simulink model "B20_ATMD_Earthquake"  (R2020b)
settings: Solver=ode45  StartTime=0.0  StopTime=30  FixedStep=Ts  MaxStep=Ts  MinStep=0.005  RelTol=1e-2
values from neighbouring files (symbols this model uses):
  DoS_on = 0    [main.m]
  EI = 0    [main.m]
  FDI_amp = 300e3    (= 300000)    [main.m]
  FDI_fr = 1/3.5104    (= 0.284867821331)    [main.m]
  FDIon = 1    [main.m]
  K_lqr = lqr(A,B,Q,R)    [main.m]
  MaxF = 2000e3    (= 2000000)    [main.m]
  nx = length(A)    [main.m]
  Sys_con = ss(A,[E B],C,D)    [main.m]
  Sys_unc = ss(A_ref,E_ref,C_ref,DD_ref)    [main.m]
  Ts = 0.01    [main.m]
  TsEarthquake = EQ.time(2)    [main.m]
undefined symbols (not defined in the file or in its folder): discount, j, So, threshold, wg2, zwg
libraries: simulink x43, dspindex x2, eeLuenbergerObserver x1
settings Model: Creator=drsoto  LastModifiedBy=ferch
settings SolverCC: AlgebraicLoopSolver=LineSearch
settings DataIOCC: ReturnWorkspaceOutputs=off
settings DebuggingCC: AlgebraicLoopMsg=none  ArithmeticOperatorsInVariantConditions=warning
settings SFSimCC: SimUseLocalCustomCode=off  CustomCodeUndefinedFunction=UseInterfaceOnly
settings RTWCC: RTWUseLocalCustomCode=off
settings CodeAppCC: StateflowObjectComments=on

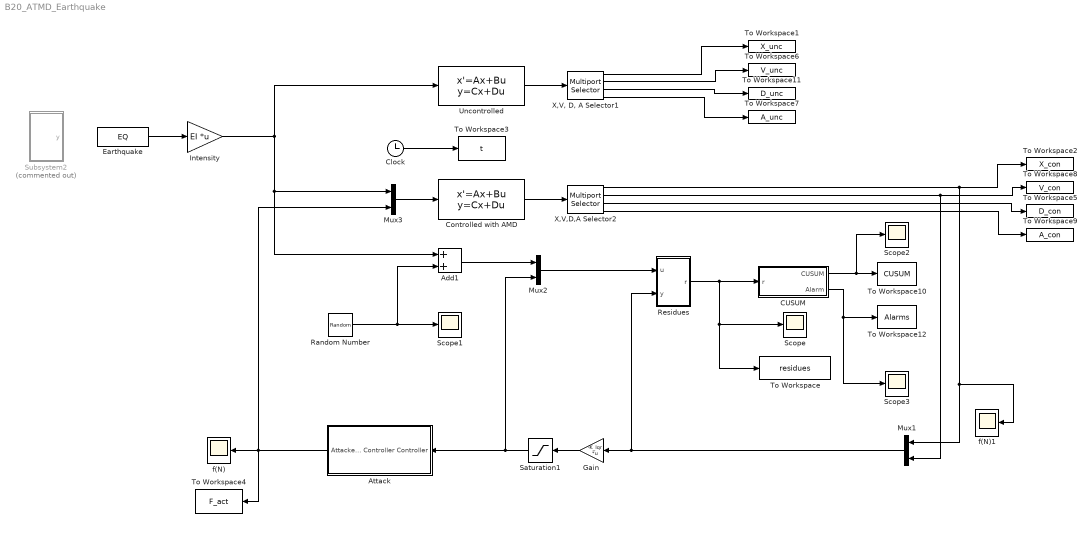
== system B20_ATMD_Earthquake ==
  Add1 : Sum
  Attack : Subsystem
  CUSUM : Subsystem
  Clock : Clock
  Controlled with AMD : StateSpace  A=Sys_con.A  B=Sys_con.B  C=Sys_con.C  D=Sys_con.D  InitialCondition=0
  Earthquake : FromWorkspace  VariableName=EQ  SampleTime=TsEarthquake
  Gain : Gain  Gain=-K_lqr  Multiplication=Matrix(K*u)
  Intensity : Gain  Gain=EI  Multiplication=Matrix(K*u)
  Mux1 : Mux  Inputs=2
  Mux2 : Mux  Inputs=2
  Mux3 : Mux  Inputs=2
  Random Number : RandomNumber  Variance=0.01  Seed=j  SampleTime=Ts
  Residues : Subsystem
  Saturation1 : Saturate  UpperLimit=MaxF  LowerLimit=-MaxF
  Scope{,1..3} (4 alike) : Scope
  Subsystem2 : Subsystem  Commented=on
  To Workspace : ToWorkspace  VariableName=residues  SaveFormat=Timeseries  SampleTime=-1
  To Workspace1 : ToWorkspace  VariableName=X_unc  SampleTime=-1
  To Workspace10 : ToWorkspace  VariableName=CUSUM  SaveFormat=Timeseries  SampleTime=-1
  To Workspace11 : ToWorkspace  VariableName=D_unc  SampleTime=-1
  To Workspace12 : ToWorkspace  VariableName=Alarms  SaveFormat=Timeseries  SampleTime=-1
  To Workspace2 : ToWorkspace  VariableName=X_con  SampleTime=-1
  To Workspace3 : ToWorkspace  VariableName=t  SampleTime=-1
      settings: Save2DSignal=2-D array (concatenate along first dimension)
  To Workspace4 : ToWorkspace  VariableName=F_act  SampleTime=-1
  To Workspace5 : ToWorkspace  VariableName=D_con  SampleTime=-1
  To Workspace6 : ToWorkspace  VariableName=V_unc  SampleTime=-1
  To Workspace7 : ToWorkspace  VariableName=A_unc  SampleTime=-1
  To Workspace8 : ToWorkspace  VariableName=V_con  SampleTime=-1
  To Workspace9 : ToWorkspace  VariableName=A_con  SampleTime=-1
  Uncontrolled : StateSpace  A=Sys_unc.A  B=Sys_unc.B  C=Sys_unc.C  D=Sys_unc.D  InitialCondition=0
  "X,V, D, A Selector1" : dspindex/Multiport Selector  rowsOrCols=Rows  idxCellArray={ 1:n,n+1:2*n,2*n+1:3*n,3*n+1:4*n}  idxErrMode=Clip Index
  X,V,D,A Selector2 : dspindex/Multiport Selector  rowsOrCols=Rows  idxCellArray={ 1:n_amd,n_amd+1:2*n_amd,2*n_amd+1:3*n_amd,3*n_amd+1:4*n_amd}  idxErrMode=Clip Index
  f(N) : Scope
  f(N)1 : Scope
  wires:
  Intensity/1 -> Uncontrolled/1, Mux3/1, Add1/1
  Uncontrolled/1 -> "X,V, D, A Selector1"/1
  Controlled with AMD/1 -> X,V,D,A Selector2/1
  Clock/1 -> To Workspace3/1
  "X,V, D, A Selector1"/2 -> To Workspace6/1
  Mux3/1 -> Controlled with AMD/1
  "X,V, D, A Selector1"/4 -> To Workspace7/1
  "X,V, D, A Selector1"/3 -> To Workspace11/1
  X,V,D,A Selector2/3 -> To Workspace5/1
  X,V,D,A Selector2/4 -> To Workspace9/1
  "X,V, D, A Selector1"/1 -> To Workspace1/1
  X,V,D,A Selector2/1 -> Mux1/1, f(N)1/1, To Workspace2/1
  X,V,D,A Selector2/2 -> To Workspace8/1, Mux1/2
  Gain/1 -> Saturation1/1
  Mux1/1 -> Residues/2(y), Gain/1
  Random Number/1 -> Scope1/1, Add1/2
  Add1/1 -> Mux2/1
  CUSUM/1(CUSUM) -> To Workspace10/1, Scope2/1
  Saturation1/1 -> Mux2/2, Attack/1(Controller)
  Residues/1(r) -> To Workspace/1, Scope/1, CUSUM/1(r)
  Mux2/1 -> Residues/1(u)
  CUSUM/2(Alarm) -> To Workspace12/1, Scope3/1
  Earthquake/1 -> Intensity/1
  Attack/1(Attacked Controller) -> Mux3/2, To Workspace4/1, f(N)/1

== system B20_ATMD_Earthquake/Attack ==
  Controller : Inport
  Constant : Constant  Value=FDIon
  Gain1 : Gain  Gain=1-DoS_on
  Saturation : Saturate  UpperLimit=MaxF  LowerLimit=-MaxF
  Sine Wave : Sin  Amplitude=FDI_amp  Frequency=FDI_fr*2*pi  SampleTime=0
  Switch : Switch  Criteria=u2 > Threshold
  Attacked Controller : Outport
  wires:
  Saturation/1 -> Gain1/1
  Controller/1 -> Switch/3
  Sine Wave/1 -> Switch/1
  Constant/1 -> Switch/2
  Switch/1 -> Saturation/1
  Gain1/1 -> Attacked Controller/1

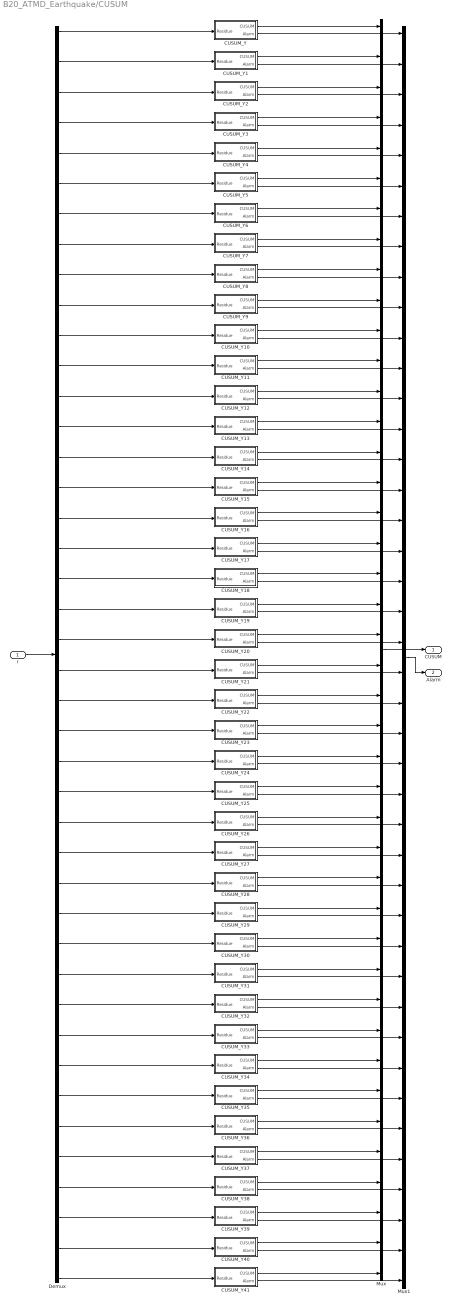
== system B20_ATMD_Earthquake/CUSUM ==
  r : Inport
  CUSUM_Y : Subsystem  mask{i=1}
      mask prompts: i "sensor"
  CUSUM_Y1 : Subsystem  mask{i=2}
      mask prompts: i "sensor"
  CUSUM_Y10 : Subsystem  mask{i=11}
      mask prompts: i "sensor"
  CUSUM_Y11 : Subsystem  mask{i=12}
      mask prompts: i "sensor"
  CUSUM_Y12 : Subsystem  mask{i=13}
      mask prompts: i "sensor"
  CUSUM_Y13 : Subsystem  mask{i=14}
      mask prompts: i "sensor"
  CUSUM_Y14 : Subsystem  mask{i=15}
      mask prompts: i "sensor"
  CUSUM_Y15 : Subsystem  mask{i=16}
      mask prompts: i "sensor"
  CUSUM_Y16 : Subsystem  mask{i=17}
      mask prompts: i "sensor"
  CUSUM_Y17 : Subsystem  mask{i=18}
      mask prompts: i "sensor"
  CUSUM_Y18 : Subsystem  mask{i=19}
      mask prompts: i "sensor"
  CUSUM_Y19 : Subsystem  mask{i=20}
      mask prompts: i "sensor"
  CUSUM_Y2 : Subsystem  mask{i=3}
      mask prompts: i "sensor"
  CUSUM_Y20 : Subsystem  mask{i=21}
      mask prompts: i "sensor"
  CUSUM_Y21 : Subsystem  mask{i=22}
      mask prompts: i "sensor"
  CUSUM_Y22 : Subsystem  mask{i=23}
      mask prompts: i "sensor"
  CUSUM_Y23 : Subsystem  mask{i=24}
      mask prompts: i "sensor"
  CUSUM_Y24 : Subsystem  mask{i=25}
      mask prompts: i "sensor"
  CUSUM_Y25 : Subsystem  mask{i=26}
      mask prompts: i "sensor"
  CUSUM_Y26 : Subsystem  mask{i=27}
      mask prompts: i "sensor"
  CUSUM_Y27 : Subsystem  mask{i=28}
      mask prompts: i "sensor"
  CUSUM_Y28 : Subsystem  mask{i=29}
      mask prompts: i "sensor"
  CUSUM_Y29 : Subsystem  mask{i=30}
      mask prompts: i "sensor"
  CUSUM_Y3 : Subsystem  mask{i=4}
      mask prompts: i "sensor"
  CUSUM_Y30 : Subsystem  mask{i=31}
      mask prompts: i "sensor"
  CUSUM_Y31 : Subsystem  mask{i=31}
      mask prompts: i "sensor"
  CUSUM_Y32 : Subsystem  mask{i=33}
      mask prompts: i "sensor"
  CUSUM_Y33 : Subsystem  mask{i=34}
      mask prompts: i "sensor"
  CUSUM_Y34 : Subsystem  mask{i=35}
      mask prompts: i "sensor"
  CUSUM_Y35 : Subsystem  mask{i=36}
      mask prompts: i "sensor"
  CUSUM_Y36 : Subsystem  mask{i=37}
      mask prompts: i "sensor"
  CUSUM_Y37 : Subsystem  mask{i=38}
      mask prompts: i "sensor"
  CUSUM_Y38 : Subsystem  mask{i=39}
      mask prompts: i "sensor"
  CUSUM_Y39 : Subsystem  mask{i=40}
      mask prompts: i "sensor"
  CUSUM_Y4 : Subsystem  mask{i=5}
      mask prompts: i "sensor"
  CUSUM_Y40 : Subsystem  mask{i=41}
      mask prompts: i "sensor"
  CUSUM_Y41 : Subsystem  mask{i=42}
      mask prompts: i "sensor"
  CUSUM_Y5 : Subsystem  mask{i=6}
      mask prompts: i "sensor"
  CUSUM_Y6 : Subsystem  mask{i=7}
      mask prompts: i "sensor"
  CUSUM_Y7 : Subsystem  mask{i=8}
      mask prompts: i "sensor"
  CUSUM_Y8 : Subsystem  mask{i=9}
      mask prompts: i "sensor"
  CUSUM_Y9 : Subsystem  mask{i=10}
      mask prompts: i "sensor"
  Demux : Demux  Outputs=42
  Mux : Mux  Inputs=42
  Mux1 : Mux  Inputs=42
  CUSUM : Outport
  Alarm : Outport  Port=2
  wires:
  r/1 -> Demux/1
  Mux/1 -> CUSUM/1
  Demux/1 -> CUSUM_Y/1(Residue)
  Demux/2 -> CUSUM_Y1/1(Residue)
  Demux/3 -> CUSUM_Y2/1(Residue)
  Demux/4 -> CUSUM_Y3/1(Residue)
  Demux/5 -> CUSUM_Y4/1(Residue)
  Demux/6 -> CUSUM_Y5/1(Residue)
  Demux/7 -> CUSUM_Y6/1(Residue)
  Demux/8 -> CUSUM_Y7/1(Residue)
  Demux/9 -> CUSUM_Y8/1(Residue)
  Demux/10 -> CUSUM_Y9/1(Residue)
  Demux/11 -> CUSUM_Y10/1(Residue)
  Demux/12 -> CUSUM_Y11/1(Residue)
  Demux/13 -> CUSUM_Y12/1(Residue)
  Demux/14 -> CUSUM_Y13/1(Residue)
  Demux/15 -> CUSUM_Y14/1(Residue)
  Demux/16 -> CUSUM_Y15/1(Residue)
  Demux/17 -> CUSUM_Y16/1(Residue)
  Demux/18 -> CUSUM_Y17/1(Residue)
  Demux/19 -> CUSUM_Y18/1(Residue)
  Demux/20 -> CUSUM_Y19/1(Residue)
  Demux/21 -> CUSUM_Y20/1(Residue)
  Demux/22 -> CUSUM_Y21/1(Residue)
  Demux/23 -> CUSUM_Y22/1(Residue)
  Demux/24 -> CUSUM_Y23/1(Residue)
  Demux/25 -> CUSUM_Y24/1(Residue)
  Demux/26 -> CUSUM_Y25/1(Residue)
  Demux/27 -> CUSUM_Y26/1(Residue)
  Demux/28 -> CUSUM_Y27/1(Residue)
  Demux/29 -> CUSUM_Y28/1(Residue)
  Demux/30 -> CUSUM_Y29/1(Residue)
  Demux/31 -> CUSUM_Y30/1(Residue)
  Demux/32 -> CUSUM_Y31/1(Residue)
  Demux/33 -> CUSUM_Y32/1(Residue)
  Demux/34 -> CUSUM_Y33/1(Residue)
  Demux/35 -> CUSUM_Y34/1(Residue)
  Demux/36 -> CUSUM_Y35/1(Residue)
  Demux/37 -> CUSUM_Y36/1(Residue)
  Demux/38 -> CUSUM_Y37/1(Residue)
  Demux/39 -> CUSUM_Y38/1(Residue)
  Demux/40 -> CUSUM_Y39/1(Residue)
  Demux/41 -> CUSUM_Y40/1(Residue)
  Demux/42 -> CUSUM_Y41/1(Residue)
  CUSUM_Y1/1(CUSUM) -> Mux/2
  CUSUM_Y/1(CUSUM) -> Mux/1
  CUSUM_Y2/1(CUSUM) -> Mux/3
  CUSUM_Y3/1(CUSUM) -> Mux/4
  CUSUM_Y4/1(CUSUM) -> Mux/5
  CUSUM_Y5/1(CUSUM) -> Mux/6
  CUSUM_Y6/1(CUSUM) -> Mux/7
  CUSUM_Y7/1(CUSUM) -> Mux/8
  CUSUM_Y8/1(CUSUM) -> Mux/9
  CUSUM_Y9/1(CUSUM) -> Mux/10
  CUSUM_Y10/1(CUSUM) -> Mux/11
  CUSUM_Y11/1(CUSUM) -> Mux/12
  CUSUM_Y12/1(CUSUM) -> Mux/13
  CUSUM_Y13/1(CUSUM) -> Mux/14
  CUSUM_Y14/1(CUSUM) -> Mux/15
  CUSUM_Y15/1(CUSUM) -> Mux/16
  CUSUM_Y16/1(CUSUM) -> Mux/17
  CUSUM_Y17/1(CUSUM) -> Mux/18
  CUSUM_Y18/1(CUSUM) -> Mux/19
  CUSUM_Y19/1(CUSUM) -> Mux/20
  CUSUM_Y20/1(CUSUM) -> Mux/21
  CUSUM_Y21/1(CUSUM) -> Mux/22
  CUSUM_Y22/1(CUSUM) -> Mux/23
  CUSUM_Y23/1(CUSUM) -> Mux/24
  CUSUM_Y24/1(CUSUM) -> Mux/25
  CUSUM_Y25/1(CUSUM) -> Mux/26
  CUSUM_Y26/1(CUSUM) -> Mux/27
  CUSUM_Y27/1(CUSUM) -> Mux/28
  CUSUM_Y28/1(CUSUM) -> Mux/29
  CUSUM_Y29/1(CUSUM) -> Mux/30
  CUSUM_Y30/1(CUSUM) -> Mux/31
  CUSUM_Y31/1(CUSUM) -> Mux/32
  CUSUM_Y32/1(CUSUM) -> Mux/33
  CUSUM_Y33/1(CUSUM) -> Mux/34
  CUSUM_Y34/1(CUSUM) -> Mux/35
  CUSUM_Y35/1(CUSUM) -> Mux/36
  CUSUM_Y36/1(CUSUM) -> Mux/37
  CUSUM_Y37/1(CUSUM) -> Mux/38
  CUSUM_Y38/1(CUSUM) -> Mux/39
  CUSUM_Y39/1(CUSUM) -> Mux/40
  CUSUM_Y40/1(CUSUM) -> Mux/41
  CUSUM_Y41/1(CUSUM) -> Mux/42
  CUSUM_Y/2(Alarm) -> Mux1/1
  CUSUM_Y1/2(Alarm) -> Mux1/2
  CUSUM_Y2/2(Alarm) -> Mux1/3
  CUSUM_Y3/2(Alarm) -> Mux1/4
  CUSUM_Y4/2(Alarm) -> Mux1/5
  CUSUM_Y5/2(Alarm) -> Mux1/6
  CUSUM_Y6/2(Alarm) -> Mux1/7
  CUSUM_Y7/2(Alarm) -> Mux1/8
  CUSUM_Y8/2(Alarm) -> Mux1/9
  CUSUM_Y9/2(Alarm) -> Mux1/10
  CUSUM_Y10/2(Alarm) -> Mux1/11
  CUSUM_Y11/2(Alarm) -> Mux1/12
  CUSUM_Y12/2(Alarm) -> Mux1/13
  CUSUM_Y13/2(Alarm) -> Mux1/14
  CUSUM_Y14/2(Alarm) -> Mux1/15
  CUSUM_Y15/2(Alarm) -> Mux1/16
  CUSUM_Y16/2(Alarm) -> Mux1/17
  CUSUM_Y17/2(Alarm) -> Mux1/18
  CUSUM_Y18/2(Alarm) -> Mux1/19
  CUSUM_Y19/2(Alarm) -> Mux1/20
  CUSUM_Y20/2(Alarm) -> Mux1/21
  CUSUM_Y21/2(Alarm) -> Mux1/22
  CUSUM_Y22/2(Alarm) -> Mux1/23
  CUSUM_Y23/2(Alarm) -> Mux1/24
  CUSUM_Y24/2(Alarm) -> Mux1/25
  CUSUM_Y25/2(Alarm) -> Mux1/26
  CUSUM_Y26/2(Alarm) -> Mux1/27
  CUSUM_Y27/2(Alarm) -> Mux1/28
  CUSUM_Y28/2(Alarm) -> Mux1/29
  CUSUM_Y29/2(Alarm) -> Mux1/30
  CUSUM_Y30/2(Alarm) -> Mux1/31
  CUSUM_Y31/2(Alarm) -> Mux1/32
  CUSUM_Y32/2(Alarm) -> Mux1/33
  CUSUM_Y33/2(Alarm) -> Mux1/34
  CUSUM_Y34/2(Alarm) -> Mux1/35
  CUSUM_Y35/2(Alarm) -> Mux1/36
  CUSUM_Y36/2(Alarm) -> Mux1/37
  CUSUM_Y37/2(Alarm) -> Mux1/38
  CUSUM_Y38/2(Alarm) -> Mux1/39
  CUSUM_Y39/2(Alarm) -> Mux1/40
  CUSUM_Y40/2(Alarm) -> Mux1/41
  CUSUM_Y41/2(Alarm) -> Mux1/42
  Mux1/1 -> Alarm/1

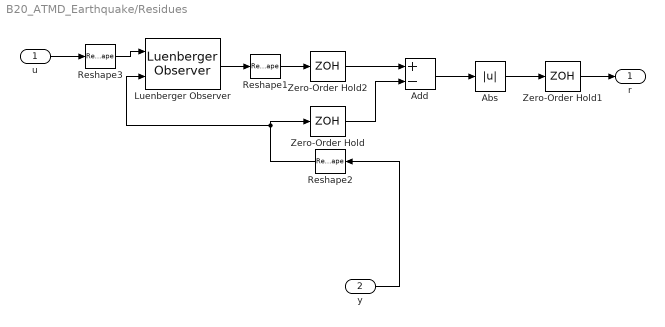
== system B20_ATMD_Earthquake/Residues ==
  u : Inport
  y : Inport  Port=2
  Abs : Abs
  Add : Sum  Inputs=+-
  Luenberger Observer : eeLuenbergerObserver/Luenberger Observer  StateSpaceType=Continuous-time  Ad=Sys_con.A  Bd=Sys_con.B  Cd=Sys_con.C  Dd=Sys_con.D  A=Sys_con.A  B=Sys_con.B  C=eye(42)  D=Sys_con.B*0  ObserverDesign=Desired eigenvalues  Ld=1  DesiredEigenvalues=[-1:-1:-nx]/5-15  x0=zeros(nx,1)  Tsd=0.1  Ts=Ts
      settings: SourceProductBaseCode=PS
  Reshape1 : Reshape
  Reshape2 : Reshape
  Reshape3 : Reshape
  Zero-Order Hold : ZeroOrderHold  SampleTime=Ts
  Zero-Order Hold1 : ZeroOrderHold  SampleTime=Ts
  Zero-Order Hold2 : ZeroOrderHold  SampleTime=Ts
  r : Outport
  wires:
  Add/1 -> Abs/1
  Luenberger Observer/1 -> Reshape1/1
  Reshape2/1 -> Zero-Order Hold/1, Luenberger Observer/2
  Reshape1/1 -> Zero-Order Hold2/1
  Zero-Order Hold2/1 -> Add/1
  Reshape3/1 -> Luenberger Observer/1
  Abs/1 -> Zero-Order Hold1/1
  Zero-Order Hold/1 -> Add/2
  y/1 -> Reshape2/1
  Zero-Order Hold1/1 -> r/1
  u/1 -> Reshape3/1

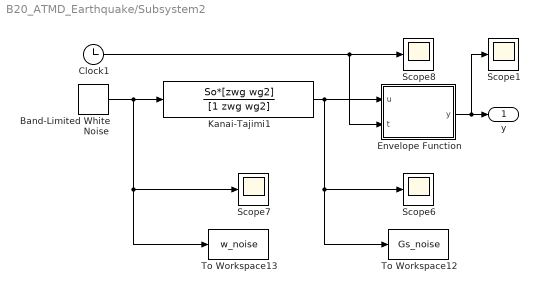
== system B20_ATMD_Earthquake/Subsystem2 ==
  Band-Limited White Noise : simulink/Sources/Band-Limited White Noise  Cov=[0.1]  Ts=Ts  seed=100
  Clock1 : Clock
  Envelope Function : MATLAB Function  TreatAsAtomicUnit=on
  Kanai-Tajimi1 : TransferFcn  Numerator=So*[zwg wg2]  Denominator=[1 zwg wg2]
  Scope{1,6..8} (4 alike) : Scope
  To Workspace12 : ToWorkspace  VariableName=Gs_noise  SampleTime=-1
  To Workspace13 : ToWorkspace  VariableName=w_noise  SampleTime=-1
  y : Outport
  wires:
  Clock1/1 -> Scope8/1, Envelope Function/2(t)
  Kanai-Tajimi1/1 -> To Workspace12/1, Scope6/1, Envelope Function/1(u)
  Band-Limited White Noise/1 -> Kanai-Tajimi1/1, Scope7/1, To Workspace13/1
  Envelope Function/1(y) -> Scope1/1, y/1

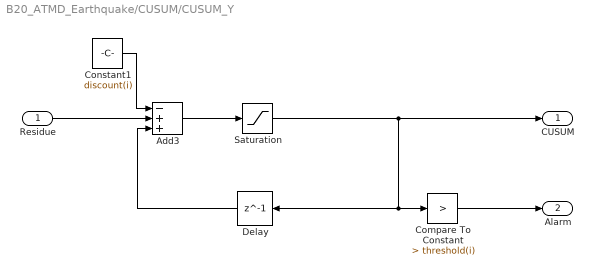
== system B20_ATMD_Earthquake/CUSUM/CUSUM_Y ==
  Residue : Inport
  Add3 : Sum  Inputs=-++
  Compare To Constant : simulink/Logic and Bit Operations/Compare To Constant  relop=>  const=threshold(i)  OutDataTypeStr=boolean
  Constant1 : Constant  Value=discount(i)
  Delay : Delay  DelayLength=1  SampleTime=Ts
  Saturation : Saturate  UpperLimit=10000  LowerLimit=0
  CUSUM : Outport  VectorParamsAs1DForOutWhenUnconnected=off
  Alarm : Outport  Port=2  VectorParamsAs1DForOutWhenUnconnected=off
  wires:
  Saturation/1 -> Compare To Constant/1, Delay/1, CUSUM/1
  Residue/1 -> Add3/2
  Delay/1 -> Add3/3
  Constant1/1 -> Add3/1
  Add3/1 -> Saturation/1
  Compare To Constant/1 -> Alarm/1

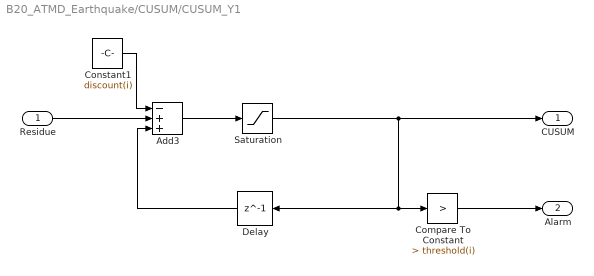
== system B20_ATMD_Earthquake/CUSUM/CUSUM_Y1 ==
  Residue : Inport
  Add3 : Sum  Inputs=-++
  Compare To Constant : simulink/Logic and Bit Operations/Compare To Constant  relop=>  const=threshold(i)  OutDataTypeStr=boolean
  Constant1 : Constant  Value=discount(i)
  Delay : Delay  DelayLength=1  SampleTime=Ts
  Saturation : Saturate  UpperLimit=10000  LowerLimit=0
  CUSUM : Outport  VectorParamsAs1DForOutWhenUnconnected=off
  Alarm : Outport  Port=2  VectorParamsAs1DForOutWhenUnconnected=off
  wires:
  Compare To Constant/1 -> Alarm/1
  Add3/1 -> Saturation/1
  Constant1/1 -> Add3/1
  Delay/1 -> Add3/3
  Residue/1 -> Add3/2
  Saturation/1 -> CUSUM/1, Delay/1, Compare To Constant/1

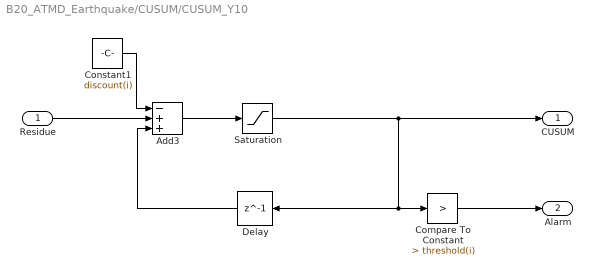
== system B20_ATMD_Earthquake/CUSUM/CUSUM_Y10 ==
  Residue : Inport
  Add3 : Sum  Inputs=-++
  Compare To Constant : simulink/Logic and Bit Operations/Compare To Constant  relop=>  const=threshold(i)  OutDataTypeStr=boolean
  Constant1 : Constant  Value=discount(i)
  Delay : Delay  DelayLength=1  SampleTime=Ts
  Saturation : Saturate  UpperLimit=10000  LowerLimit=0
  CUSUM : Outport  VectorParamsAs1DForOutWhenUnconnected=off
  Alarm : Outport  Port=2  VectorParamsAs1DForOutWhenUnconnected=off
  wires:
  Compare To Constant/1 -> Alarm/1
  Add3/1 -> Saturation/1
  Constant1/1 -> Add3/1
  Delay/1 -> Add3/3
  Residue/1 -> Add3/2
  Saturation/1 -> CUSUM/1, Delay/1, Compare To Constant/1

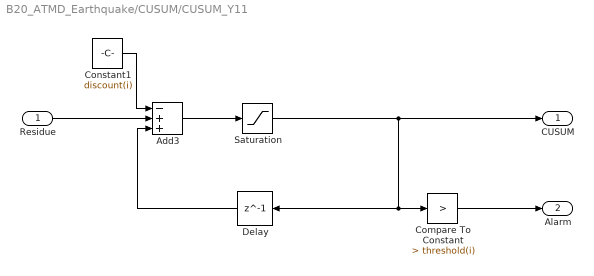
== system B20_ATMD_Earthquake/CUSUM/CUSUM_Y11 ==
  Residue : Inport
  Add3 : Sum  Inputs=-++
  Compare To Constant : simulink/Logic and Bit Operations/Compare To Constant  relop=>  const=threshold(i)  OutDataTypeStr=boolean
  Constant1 : Constant  Value=discount(i)
  Delay : Delay  DelayLength=1  SampleTime=Ts
  Saturation : Saturate  UpperLimit=10000  LowerLimit=0
  CUSUM : Outport  VectorParamsAs1DForOutWhenUnconnected=off
  Alarm : Outport  Port=2  VectorParamsAs1DForOutWhenUnconnected=off
  wires:
  Saturation/1 -> Compare To Constant/1, Delay/1, CUSUM/1
  Residue/1 -> Add3/2
  Delay/1 -> Add3/3
  Constant1/1 -> Add3/1
  Add3/1 -> Saturation/1
  Compare To Constant/1 -> Alarm/1

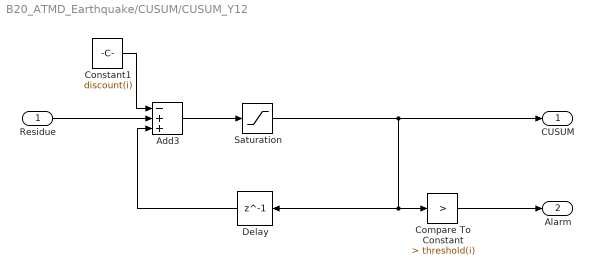
== system B20_ATMD_Earthquake/CUSUM/CUSUM_Y12 ==
  Residue : Inport
  Add3 : Sum  Inputs=-++
  Compare To Constant : simulink/Logic and Bit Operations/Compare To Constant  relop=>  const=threshold(i)  OutDataTypeStr=boolean
  Constant1 : Constant  Value=discount(i)
  Delay : Delay  DelayLength=1  SampleTime=Ts
  Saturation : Saturate  UpperLimit=10000  LowerLimit=0
  CUSUM : Outport  VectorParamsAs1DForOutWhenUnconnected=off
  Alarm : Outport  Port=2  VectorParamsAs1DForOutWhenUnconnected=off
  wires:
  Saturation/1 -> Compare To Constant/1, Delay/1, CUSUM/1
  Residue/1 -> Add3/2
  Delay/1 -> Add3/3
  Constant1/1 -> Add3/1
  Add3/1 -> Saturation/1
  Compare To Constant/1 -> Alarm/1

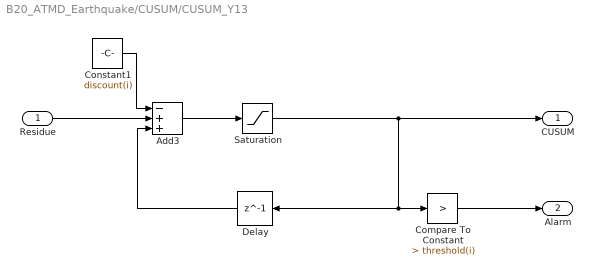
== system B20_ATMD_Earthquake/CUSUM/CUSUM_Y13 ==
  Residue : Inport
  Add3 : Sum  Inputs=-++
  Compare To Constant : simulink/Logic and Bit Operations/Compare To Constant  relop=>  const=threshold(i)  OutDataTypeStr=boolean
  Constant1 : Constant  Value=discount(i)
  Delay : Delay  DelayLength=1  SampleTime=Ts
  Saturation : Saturate  UpperLimit=10000  LowerLimit=0
  CUSUM : Outport  VectorParamsAs1DForOutWhenUnconnected=off
  Alarm : Outport  Port=2  VectorParamsAs1DForOutWhenUnconnected=off
  wires:
  Compare To Constant/1 -> Alarm/1
  Add3/1 -> Saturation/1
  Constant1/1 -> Add3/1
  Delay/1 -> Add3/3
  Residue/1 -> Add3/2
  Saturation/1 -> CUSUM/1, Delay/1, Compare To Constant/1

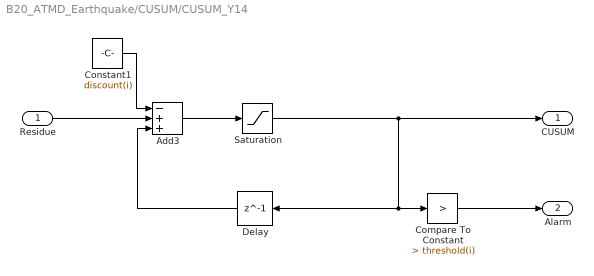
== system B20_ATMD_Earthquake/CUSUM/CUSUM_Y14 ==
  Residue : Inport
  Add3 : Sum  Inputs=-++
  Compare To Constant : simulink/Logic and Bit Operations/Compare To Constant  relop=>  const=threshold(i)  OutDataTypeStr=boolean
  Constant1 : Constant  Value=discount(i)
  Delay : Delay  DelayLength=1  SampleTime=Ts
  Saturation : Saturate  UpperLimit=10000  LowerLimit=0
  CUSUM : Outport  VectorParamsAs1DForOutWhenUnconnected=off
  Alarm : Outport  Port=2  VectorParamsAs1DForOutWhenUnconnected=off
  wires:
  Compare To Constant/1 -> Alarm/1
  Add3/1 -> Saturation/1
  Constant1/1 -> Add3/1
  Delay/1 -> Add3/3
  Residue/1 -> Add3/2
  Saturation/1 -> CUSUM/1, Delay/1, Compare To Constant/1

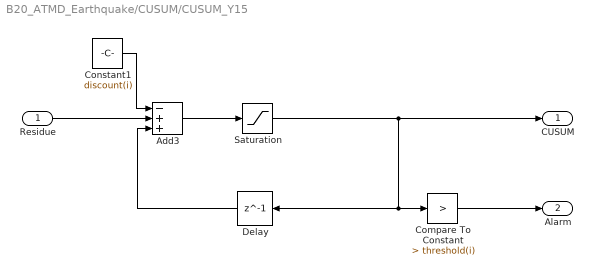
== system B20_ATMD_Earthquake/CUSUM/CUSUM_Y15 ==
  Residue : Inport
  Add3 : Sum  Inputs=-++
  Compare To Constant : simulink/Logic and Bit Operations/Compare To Constant  relop=>  const=threshold(i)  OutDataTypeStr=boolean
  Constant1 : Constant  Value=discount(i)
  Delay : Delay  DelayLength=1  SampleTime=Ts
  Saturation : Saturate  UpperLimit=10000  LowerLimit=0
  CUSUM : Outport  VectorParamsAs1DForOutWhenUnconnected=off
  Alarm : Outport  Port=2  VectorParamsAs1DForOutWhenUnconnected=off
  wires:
  Saturation/1 -> Compare To Constant/1, Delay/1, CUSUM/1
  Residue/1 -> Add3/2
  Delay/1 -> Add3/3
  Constant1/1 -> Add3/1
  Add3/1 -> Saturation/1
  Compare To Constant/1 -> Alarm/1

== system B20_ATMD_Earthquake/CUSUM/CUSUM_Y16 ==
  Residue : Inport
  Add3 : Sum  Inputs=-++
  Compare To Constant : simulink/Logic and Bit Operations/Compare To Constant  relop=>  const=threshold(i)  OutDataTypeStr=boolean
  Constant1 : Constant  Value=discount(i)
  Delay : Delay  DelayLength=1  SampleTime=Ts
  Saturation : Saturate  UpperLimit=10000  LowerLimit=0
  CUSUM : Outport  VectorParamsAs1DForOutWhenUnconnected=off
  Alarm : Outport  Port=2  VectorParamsAs1DForOutWhenUnconnected=off
  wires:
  Saturation/1 -> Compare To Constant/1, Delay/1, CUSUM/1
  Residue/1 -> Add3/2
  Delay/1 -> Add3/3
  Constant1/1 -> Add3/1
  Add3/1 -> Saturation/1
  Compare To Constant/1 -> Alarm/1

== system B20_ATMD_Earthquake/CUSUM/CUSUM_Y17 ==
  Residue : Inport
  Add3 : Sum  Inputs=-++
  Compare To Constant : simulink/Logic and Bit Operations/Compare To Constant  relop=>  const=threshold(i)  OutDataTypeStr=boolean
  Constant1 : Constant  Value=discount(i)
  Delay : Delay  DelayLength=1  SampleTime=Ts
  Saturation : Saturate  UpperLimit=10000  LowerLimit=0
  CUSUM : Outport  VectorParamsAs1DForOutWhenUnconnected=off
  Alarm : Outport  Port=2  VectorParamsAs1DForOutWhenUnconnected=off
  wires:
  Compare To Constant/1 -> Alarm/1
  Add3/1 -> Saturation/1
  Constant1/1 -> Add3/1
  Delay/1 -> Add3/3
  Residue/1 -> Add3/2
  Saturation/1 -> CUSUM/1, Delay/1, Compare To Constant/1

== system B20_ATMD_Earthquake/CUSUM/CUSUM_Y18 ==
  Residue : Inport
  Add3 : Sum  Inputs=-++
  Compare To Constant : simulink/Logic and Bit Operations/Compare To Constant  relop=>  const=threshold(i)  OutDataTypeStr=boolean
  Constant1 : Constant  Value=discount(i)
  Delay : Delay  DelayLength=1  SampleTime=Ts
  Saturation : Saturate  UpperLimit=10000  LowerLimit=0
  CUSUM : Outport  VectorParamsAs1DForOutWhenUnconnected=off
  Alarm : Outport  Port=2  VectorParamsAs1DForOutWhenUnconnected=off
  wires:
  Compare To Constant/1 -> Alarm/1
  Add3/1 -> Saturation/1
  Constant1/1 -> Add3/1
  Delay/1 -> Add3/3
  Residue/1 -> Add3/2
  Saturation/1 -> CUSUM/1, Delay/1, Compare To Constant/1

== system B20_ATMD_Earthquake/CUSUM/CUSUM_Y19 ==
  Residue : Inport
  Add3 : Sum  Inputs=-++
  Compare To Constant : simulink/Logic and Bit Operations/Compare To Constant  relop=>  const=threshold(i)  OutDataTypeStr=boolean
  Constant1 : Constant  Value=discount(i)
  Delay : Delay  DelayLength=1  SampleTime=Ts
  Saturation : Saturate  UpperLimit=10000  LowerLimit=0
  CUSUM : Outport  VectorParamsAs1DForOutWhenUnconnected=off
  Alarm : Outport  Port=2  VectorParamsAs1DForOutWhenUnconnected=off
  wires:
  Saturation/1 -> Compare To Constant/1, Delay/1, CUSUM/1
  Residue/1 -> Add3/2
  Delay/1 -> Add3/3
  Constant1/1 -> Add3/1
  Add3/1 -> Saturation/1
  Compare To Constant/1 -> Alarm/1

== system B20_ATMD_Earthquake/CUSUM/CUSUM_Y2 ==
  Residue : Inport
  Add3 : Sum  Inputs=-++
  Compare To Constant : simulink/Logic and Bit Operations/Compare To Constant  relop=>  const=threshold(i)  OutDataTypeStr=boolean
  Constant1 : Constant  Value=discount(i)
  Delay : Delay  DelayLength=1  SampleTime=Ts
  Saturation : Saturate  UpperLimit=10000  LowerLimit=0
  CUSUM : Outport  VectorParamsAs1DForOutWhenUnconnected=off
  Alarm : Outport  Port=2  VectorParamsAs1DForOutWhenUnconnected=off
  wires:
  Compare To Constant/1 -> Alarm/1
  Add3/1 -> Saturation/1
  Constant1/1 -> Add3/1
  Delay/1 -> Add3/3
  Residue/1 -> Add3/2
  Saturation/1 -> CUSUM/1, Delay/1, Compare To Constant/1

== system B20_ATMD_Earthquake/CUSUM/CUSUM_Y20 ==
  Residue : Inport
  Add3 : Sum  Inputs=-++
  Compare To Constant : simulink/Logic and Bit Operations/Compare To Constant  relop=>  const=threshold(i)  OutDataTypeStr=boolean
  Constant1 : Constant  Value=discount(i)
  Delay : Delay  DelayLength=1  SampleTime=Ts
  Saturation : Saturate  UpperLimit=10000  LowerLimit=0
  CUSUM : Outport  VectorParamsAs1DForOutWhenUnconnected=off
  Alarm : Outport  Port=2  VectorParamsAs1DForOutWhenUnconnected=off
  wires:
  Saturation/1 -> Compare To Constant/1, Delay/1, CUSUM/1
  Residue/1 -> Add3/2
  Delay/1 -> Add3/3
  Constant1/1 -> Add3/1
  Add3/1 -> Saturation/1
  Compare To Constant/1 -> Alarm/1

== system B20_ATMD_Earthquake/CUSUM/CUSUM_Y21 ==
  Residue : Inport
  Add3 : Sum  Inputs=-++
  Compare To Constant : simulink/Logic and Bit Operations/Compare To Constant  relop=>  const=threshold(i)  OutDataTypeStr=boolean
  Constant1 : Constant  Value=discount(i)
  Delay : Delay  DelayLength=1  SampleTime=Ts
  Saturation : Saturate  UpperLimit=10000  LowerLimit=0
  CUSUM : Outport  VectorParamsAs1DForOutWhenUnconnected=off
  Alarm : Outport  Port=2  VectorParamsAs1DForOutWhenUnconnected=off
  wires:
  Saturation/1 -> Compare To Constant/1, Delay/1, CUSUM/1
  Residue/1 -> Add3/2
  Delay/1 -> Add3/3
  Constant1/1 -> Add3/1
  Add3/1 -> Saturation/1
  Compare To Constant/1 -> Alarm/1

== system B20_ATMD_Earthquake/CUSUM/CUSUM_Y22 ==
  Residue : Inport
  Add3 : Sum  Inputs=-++
  Compare To Constant : simulink/Logic and Bit Operations/Compare To Constant  relop=>  const=threshold(i)  OutDataTypeStr=boolean
  Constant1 : Constant  Value=discount(i)
  Delay : Delay  DelayLength=1  SampleTime=Ts
  Saturation : Saturate  UpperLimit=10000  LowerLimit=0
  CUSUM : Outport  VectorParamsAs1DForOutWhenUnconnected=off
  Alarm : Outport  Port=2  VectorParamsAs1DForOutWhenUnconnected=off
  wires:
  Compare To Constant/1 -> Alarm/1
  Add3/1 -> Saturation/1
  Constant1/1 -> Add3/1
  Delay/1 -> Add3/3
  Residue/1 -> Add3/2
  Saturation/1 -> CUSUM/1, Delay/1, Compare To Constant/1

== system B20_ATMD_Earthquake/CUSUM/CUSUM_Y23 ==
  Residue : Inport
  Add3 : Sum  Inputs=-++
  Compare To Constant : simulink/Logic and Bit Operations/Compare To Constant  relop=>  const=threshold(i)  OutDataTypeStr=boolean
  Constant1 : Constant  Value=discount(i)
  Delay : Delay  DelayLength=1  SampleTime=Ts
  Saturation : Saturate  UpperLimit=10000  LowerLimit=0
  CUSUM : Outport  VectorParamsAs1DForOutWhenUnconnected=off
  Alarm : Outport  Port=2  VectorParamsAs1DForOutWhenUnconnected=off
  wires:
  Compare To Constant/1 -> Alarm/1
  Add3/1 -> Saturation/1
  Constant1/1 -> Add3/1
  Delay/1 -> Add3/3
  Residue/1 -> Add3/2
  Saturation/1 -> CUSUM/1, Delay/1, Compare To Constant/1

== system B20_ATMD_Earthquake/CUSUM/CUSUM_Y24 ==
  Residue : Inport
  Add3 : Sum  Inputs=-++
  Compare To Constant : simulink/Logic and Bit Operations/Compare To Constant  relop=>  const=threshold(i)  OutDataTypeStr=boolean
  Constant1 : Constant  Value=discount(i)
  Delay : Delay  DelayLength=1  SampleTime=Ts
  Saturation : Saturate  UpperLimit=10000  LowerLimit=0
  CUSUM : Outport  VectorParamsAs1DForOutWhenUnconnected=off
  Alarm : Outport  Port=2  VectorParamsAs1DForOutWhenUnconnected=off
  wires:
  Saturation/1 -> Compare To Constant/1, Delay/1, CUSUM/1
  Residue/1 -> Add3/2
  Delay/1 -> Add3/3
  Constant1/1 -> Add3/1
  Add3/1 -> Saturation/1
  Compare To Constant/1 -> Alarm/1

== system B20_ATMD_Earthquake/CUSUM/CUSUM_Y25 ==
  Residue : Inport
  Add3 : Sum  Inputs=-++
  Compare To Constant : simulink/Logic and Bit Operations/Compare To Constant  relop=>  const=threshold(i)  OutDataTypeStr=boolean
  Constant1 : Constant  Value=discount(i)
  Delay : Delay  DelayLength=1  SampleTime=Ts
  Saturation : Saturate  UpperLimit=10000  LowerLimit=0
  CUSUM : Outport  VectorParamsAs1DForOutWhenUnconnected=off
  Alarm : Outport  Port=2  VectorParamsAs1DForOutWhenUnconnected=off
  wires:
  Saturation/1 -> Compare To Constant/1, Delay/1, CUSUM/1
  Residue/1 -> Add3/2
  Delay/1 -> Add3/3
  Constant1/1 -> Add3/1
  Add3/1 -> Saturation/1
  Compare To Constant/1 -> Alarm/1

== system B20_ATMD_Earthquake/CUSUM/CUSUM_Y26 ==
  Residue : Inport
  Add3 : Sum  Inputs=-++
  Compare To Constant : simulink/Logic and Bit Operations/Compare To Constant  relop=>  const=threshold(i)  OutDataTypeStr=boolean
  Constant1 : Constant  Value=discount(i)
  Delay : Delay  DelayLength=1  SampleTime=Ts
  Saturation : Saturate  UpperLimit=10000  LowerLimit=0
  CUSUM : Outport  VectorParamsAs1DForOutWhenUnconnected=off
  Alarm : Outport  Port=2  VectorParamsAs1DForOutWhenUnconnected=off
  wires:
  Saturation/1 -> Compare To Constant/1, Delay/1, CUSUM/1
  Residue/1 -> Add3/2
  Delay/1 -> Add3/3
  Constant1/1 -> Add3/1
  Add3/1 -> Saturation/1
  Compare To Constant/1 -> Alarm/1

== system B20_ATMD_Earthquake/CUSUM/CUSUM_Y27 ==
  Residue : Inport
  Add3 : Sum  Inputs=-++
  Compare To Constant : simulink/Logic and Bit Operations/Compare To Constant  relop=>  const=threshold(i)  OutDataTypeStr=boolean
  Constant1 : Constant  Value=discount(i)
  Delay : Delay  DelayLength=1  SampleTime=Ts
  Saturation : Saturate  UpperLimit=10000  LowerLimit=0
  CUSUM : Outport  VectorParamsAs1DForOutWhenUnconnected=off
  Alarm : Outport  Port=2  VectorParamsAs1DForOutWhenUnconnected=off
  wires:
  Compare To Constant/1 -> Alarm/1
  Add3/1 -> Saturation/1
  Constant1/1 -> Add3/1
  Delay/1 -> Add3/3
  Residue/1 -> Add3/2
  Saturation/1 -> CUSUM/1, Delay/1, Compare To Constant/1

== system B20_ATMD_Earthquake/CUSUM/CUSUM_Y28 ==
  Residue : Inport
  Add3 : Sum  Inputs=-++
  Compare To Constant : simulink/Logic and Bit Operations/Compare To Constant  relop=>  const=threshold(i)  OutDataTypeStr=boolean
  Constant1 : Constant  Value=discount(i)
  Delay : Delay  DelayLength=1  SampleTime=Ts
  Saturation : Saturate  UpperLimit=10000  LowerLimit=0
  CUSUM : Outport  VectorParamsAs1DForOutWhenUnconnected=off
  Alarm : Outport  Port=2  VectorParamsAs1DForOutWhenUnconnected=off
  wires:
  Compare To Constant/1 -> Alarm/1
  Add3/1 -> Saturation/1
  Constant1/1 -> Add3/1
  Delay/1 -> Add3/3
  Residue/1 -> Add3/2
  Saturation/1 -> CUSUM/1, Delay/1, Compare To Constant/1

== system B20_ATMD_Earthquake/CUSUM/CUSUM_Y29 ==
  Residue : Inport
  Add3 : Sum  Inputs=-++
  Compare To Constant : simulink/Logic and Bit Operations/Compare To Constant  relop=>  const=threshold(i)  OutDataTypeStr=boolean
  Constant1 : Constant  Value=discount(i)
  Delay : Delay  DelayLength=1  SampleTime=Ts
  Saturation : Saturate  UpperLimit=10000  LowerLimit=0
  CUSUM : Outport  VectorParamsAs1DForOutWhenUnconnected=off
  Alarm : Outport  Port=2  VectorParamsAs1DForOutWhenUnconnected=off
  wires:
  Saturation/1 -> Compare To Constant/1, Delay/1, CUSUM/1
  Residue/1 -> Add3/2
  Delay/1 -> Add3/3
  Constant1/1 -> Add3/1
  Add3/1 -> Saturation/1
  Compare To Constant/1 -> Alarm/1

== system B20_ATMD_Earthquake/CUSUM/CUSUM_Y3 ==
  Residue : Inport
  Add3 : Sum  Inputs=-++
  Compare To Constant : simulink/Logic and Bit Operations/Compare To Constant  relop=>  const=threshold(i)  OutDataTypeStr=boolean
  Constant1 : Constant  Value=discount(i)
  Delay : Delay  DelayLength=1  SampleTime=Ts
  Saturation : Saturate  UpperLimit=10000  LowerLimit=0
  CUSUM : Outport  VectorParamsAs1DForOutWhenUnconnected=off
  Alarm : Outport  Port=2  VectorParamsAs1DForOutWhenUnconnected=off
  wires:
  Saturation/1 -> Compare To Constant/1, Delay/1, CUSUM/1
  Residue/1 -> Add3/2
  Delay/1 -> Add3/3
  Constant1/1 -> Add3/1
  Add3/1 -> Saturation/1
  Compare To Constant/1 -> Alarm/1

== system B20_ATMD_Earthquake/CUSUM/CUSUM_Y30 ==
  Residue : Inport
  Add3 : Sum  Inputs=-++
  Compare To Constant : simulink/Logic and Bit Operations/Compare To Constant  relop=>  const=threshold(i)  OutDataTypeStr=boolean
  Constant1 : Constant  Value=discount(i)
  Delay : Delay  DelayLength=1  SampleTime=Ts
  Saturation : Saturate  UpperLimit=10000  LowerLimit=0
  CUSUM : Outport  VectorParamsAs1DForOutWhenUnconnected=off
  Alarm : Outport  Port=2  VectorParamsAs1DForOutWhenUnconnected=off
  wires:
  Saturation/1 -> Compare To Constant/1, Delay/1, CUSUM/1
  Residue/1 -> Add3/2
  Delay/1 -> Add3/3
  Constant1/1 -> Add3/1
  Add3/1 -> Saturation/1
  Compare To Constant/1 -> Alarm/1

== system B20_ATMD_Earthquake/CUSUM/CUSUM_Y31 ==
  Residue : Inport
  Add3 : Sum  Inputs=-++
  Compare To Constant : simulink/Logic and Bit Operations/Compare To Constant  relop=>  const=threshold(i)  OutDataTypeStr=boolean
  Constant1 : Constant  Value=discount(i)
  Delay : Delay  DelayLength=1  SampleTime=Ts
  Saturation : Saturate  UpperLimit=10000  LowerLimit=0
  CUSUM : Outport  VectorParamsAs1DForOutWhenUnconnected=off
  Alarm : Outport  Port=2  VectorParamsAs1DForOutWhenUnconnected=off
  wires:
  Saturation/1 -> Compare To Constant/1, Delay/1, CUSUM/1
  Residue/1 -> Add3/2
  Delay/1 -> Add3/3
  Constant1/1 -> Add3/1
  Add3/1 -> Saturation/1
  Compare To Constant/1 -> Alarm/1

== system B20_ATMD_Earthquake/CUSUM/CUSUM_Y32 ==
  Residue : Inport
  Add3 : Sum  Inputs=-++
  Compare To Constant : simulink/Logic and Bit Operations/Compare To Constant  relop=>  const=threshold(i)  OutDataTypeStr=boolean
  Constant1 : Constant  Value=discount(i)
  Delay : Delay  DelayLength=1  SampleTime=Ts
  Saturation : Saturate  UpperLimit=10000  LowerLimit=0
  CUSUM : Outport  VectorParamsAs1DForOutWhenUnconnected=off
  Alarm : Outport  Port=2  VectorParamsAs1DForOutWhenUnconnected=off
  wires:
  Compare To Constant/1 -> Alarm/1
  Add3/1 -> Saturation/1
  Constant1/1 -> Add3/1
  Delay/1 -> Add3/3
  Residue/1 -> Add3/2
  Saturation/1 -> CUSUM/1, Delay/1, Compare To Constant/1

== system B20_ATMD_Earthquake/CUSUM/CUSUM_Y33 ==
  Residue : Inport
  Add3 : Sum  Inputs=-++
  Compare To Constant : simulink/Logic and Bit Operations/Compare To Constant  relop=>  const=threshold(i)  OutDataTypeStr=boolean
  Constant1 : Constant  Value=discount(i)
  Delay : Delay  DelayLength=1  SampleTime=Ts
  Saturation : Saturate  UpperLimit=10000  LowerLimit=0
  CUSUM : Outport  VectorParamsAs1DForOutWhenUnconnected=off
  Alarm : Outport  Port=2  VectorParamsAs1DForOutWhenUnconnected=off
  wires:
  Compare To Constant/1 -> Alarm/1
  Add3/1 -> Saturation/1
  Constant1/1 -> Add3/1
  Delay/1 -> Add3/3
  Residue/1 -> Add3/2
  Saturation/1 -> CUSUM/1, Delay/1, Compare To Constant/1

== system B20_ATMD_Earthquake/CUSUM/CUSUM_Y34 ==
  Residue : Inport
  Add3 : Sum  Inputs=-++
  Compare To Constant : simulink/Logic and Bit Operations/Compare To Constant  relop=>  const=threshold(i)  OutDataTypeStr=boolean
  Constant1 : Constant  Value=discount(i)
  Delay : Delay  DelayLength=1  SampleTime=Ts
  Saturation : Saturate  UpperLimit=10000  LowerLimit=0
  CUSUM : Outport  VectorParamsAs1DForOutWhenUnconnected=off
  Alarm : Outport  Port=2  VectorParamsAs1DForOutWhenUnconnected=off
  wires:
  Saturation/1 -> Compare To Constant/1, Delay/1, CUSUM/1
  Residue/1 -> Add3/2
  Delay/1 -> Add3/3
  Constant1/1 -> Add3/1
  Add3/1 -> Saturation/1
  Compare To Constant/1 -> Alarm/1

== system B20_ATMD_Earthquake/CUSUM/CUSUM_Y35 ==
  Residue : Inport
  Add3 : Sum  Inputs=-++
  Compare To Constant : simulink/Logic and Bit Operations/Compare To Constant  relop=>  const=threshold(i)  OutDataTypeStr=boolean
  Constant1 : Constant  Value=discount(i)
  Delay : Delay  DelayLength=1  SampleTime=Ts
  Saturation : Saturate  UpperLimit=10000  LowerLimit=0
  CUSUM : Outport  VectorParamsAs1DForOutWhenUnconnected=off
  Alarm : Outport  Port=2  VectorParamsAs1DForOutWhenUnconnected=off
  wires:
  Compare To Constant/1 -> Alarm/1
  Add3/1 -> Saturation/1
  Constant1/1 -> Add3/1
  Delay/1 -> Add3/3
  Residue/1 -> Add3/2
  Saturation/1 -> CUSUM/1, Delay/1, Compare To Constant/1

== system B20_ATMD_Earthquake/CUSUM/CUSUM_Y36 ==
  Residue : Inport
  Add3 : Sum  Inputs=-++
  Compare To Constant : simulink/Logic and Bit Operations/Compare To Constant  relop=>  const=threshold(i)  OutDataTypeStr=boolean
  Constant1 : Constant  Value=discount(i)
  Delay : Delay  DelayLength=1  SampleTime=Ts
  Saturation : Saturate  UpperLimit=10000  LowerLimit=0
  CUSUM : Outport  VectorParamsAs1DForOutWhenUnconnected=off
  Alarm : Outport  Port=2  VectorParamsAs1DForOutWhenUnconnected=off
  wires:
  Saturation/1 -> Compare To Constant/1, Delay/1, CUSUM/1
  Residue/1 -> Add3/2
  Delay/1 -> Add3/3
  Constant1/1 -> Add3/1
  Add3/1 -> Saturation/1
  Compare To Constant/1 -> Alarm/1

== system B20_ATMD_Earthquake/CUSUM/CUSUM_Y37 ==
  Residue : Inport
  Add3 : Sum  Inputs=-++
  Compare To Constant : simulink/Logic and Bit Operations/Compare To Constant  relop=>  const=threshold(i)  OutDataTypeStr=boolean
  Constant1 : Constant  Value=discount(i)
  Delay : Delay  DelayLength=1  SampleTime=Ts
  Saturation : Saturate  UpperLimit=10000  LowerLimit=0
  CUSUM : Outport  VectorParamsAs1DForOutWhenUnconnected=off
  Alarm : Outport  Port=2  VectorParamsAs1DForOutWhenUnconnected=off
  wires:
  Saturation/1 -> Compare To Constant/1, Delay/1, CUSUM/1
  Residue/1 -> Add3/2
  Delay/1 -> Add3/3
  Constant1/1 -> Add3/1
  Add3/1 -> Saturation/1
  Compare To Constant/1 -> Alarm/1

== system B20_ATMD_Earthquake/CUSUM/CUSUM_Y38 ==
  Residue : Inport
  Add3 : Sum  Inputs=-++
  Compare To Constant : simulink/Logic and Bit Operations/Compare To Constant  relop=>  const=threshold(i)  OutDataTypeStr=boolean
  Constant1 : Constant  Value=discount(i)
  Delay : Delay  DelayLength=1  SampleTime=Ts
  Saturation : Saturate  UpperLimit=10000  LowerLimit=0
  CUSUM : Outport  VectorParamsAs1DForOutWhenUnconnected=off
  Alarm : Outport  Port=2  VectorParamsAs1DForOutWhenUnconnected=off
  wires:
  Saturation/1 -> Compare To Constant/1, Delay/1, CUSUM/1
  Residue/1 -> Add3/2
  Delay/1 -> Add3/3
  Constant1/1 -> Add3/1
  Add3/1 -> Saturation/1
  Compare To Constant/1 -> Alarm/1

== system B20_ATMD_Earthquake/CUSUM/CUSUM_Y39 ==
  Residue : Inport
  Add3 : Sum  Inputs=-++
  Compare To Constant : simulink/Logic and Bit Operations/Compare To Constant  relop=>  const=threshold(i)  OutDataTypeStr=boolean
  Constant1 : Constant  Value=discount(i)
  Delay : Delay  DelayLength=1  SampleTime=Ts
  Saturation : Saturate  UpperLimit=10000  LowerLimit=0
  CUSUM : Outport  VectorParamsAs1DForOutWhenUnconnected=off
  Alarm : Outport  Port=2  VectorParamsAs1DForOutWhenUnconnected=off
  wires:
  Compare To Constant/1 -> Alarm/1
  Add3/1 -> Saturation/1
  Constant1/1 -> Add3/1
  Delay/1 -> Add3/3
  Residue/1 -> Add3/2
  Saturation/1 -> CUSUM/1, Delay/1, Compare To Constant/1

== system B20_ATMD_Earthquake/CUSUM/CUSUM_Y4 ==
  Residue : Inport
  Add3 : Sum  Inputs=-++
  Compare To Constant : simulink/Logic and Bit Operations/Compare To Constant  relop=>  const=threshold(i)  OutDataTypeStr=boolean
  Constant1 : Constant  Value=discount(i)
  Delay : Delay  DelayLength=1  SampleTime=Ts
  Saturation : Saturate  UpperLimit=10000  LowerLimit=0
  CUSUM : Outport  VectorParamsAs1DForOutWhenUnconnected=off
  Alarm : Outport  Port=2  VectorParamsAs1DForOutWhenUnconnected=off
  wires:
  Saturation/1 -> Compare To Constant/1, Delay/1, CUSUM/1
  Residue/1 -> Add3/2
  Delay/1 -> Add3/3
  Constant1/1 -> Add3/1
  Add3/1 -> Saturation/1
  Compare To Constant/1 -> Alarm/1

== system B20_ATMD_Earthquake/CUSUM/CUSUM_Y40 ==
  Residue : Inport
  Add3 : Sum  Inputs=-++
  Compare To Constant : simulink/Logic and Bit Operations/Compare To Constant  relop=>  const=threshold(i)  OutDataTypeStr=boolean
  Constant1 : Constant  Value=discount(i)
  Delay : Delay  DelayLength=1  SampleTime=Ts
  Saturation : Saturate  UpperLimit=10000  LowerLimit=0
  CUSUM : Outport  VectorParamsAs1DForOutWhenUnconnected=off
  Alarm : Outport  Port=2  VectorParamsAs1DForOutWhenUnconnected=off
  wires:
  Compare To Constant/1 -> Alarm/1
  Add3/1 -> Saturation/1
  Constant1/1 -> Add3/1
  Delay/1 -> Add3/3
  Residue/1 -> Add3/2
  Saturation/1 -> CUSUM/1, Delay/1, Compare To Constant/1

== system B20_ATMD_Earthquake/CUSUM/CUSUM_Y41 ==
  Residue : Inport
  Add3 : Sum  Inputs=-++
  Compare To Constant : simulink/Logic and Bit Operations/Compare To Constant  relop=>  const=threshold(i)  OutDataTypeStr=boolean
  Constant1 : Constant  Value=discount(i)
  Delay : Delay  DelayLength=1  SampleTime=Ts
  Saturation : Saturate  UpperLimit=10000  LowerLimit=0
  CUSUM : Outport  VectorParamsAs1DForOutWhenUnconnected=off
  Alarm : Outport  Port=2  VectorParamsAs1DForOutWhenUnconnected=off
  wires:
  Saturation/1 -> Compare To Constant/1, Delay/1, CUSUM/1
  Residue/1 -> Add3/2
  Delay/1 -> Add3/3
  Constant1/1 -> Add3/1
  Add3/1 -> Saturation/1
  Compare To Constant/1 -> Alarm/1

== system B20_ATMD_Earthquake/CUSUM/CUSUM_Y5 ==
  Residue : Inport
  Add3 : Sum  Inputs=-++
  Compare To Constant : simulink/Logic and Bit Operations/Compare To Constant  relop=>  const=threshold(i)  OutDataTypeStr=boolean
  Constant1 : Constant  Value=discount(i)
  Delay : Delay  DelayLength=1  SampleTime=Ts
  Saturation : Saturate  UpperLimit=10000  LowerLimit=0
  CUSUM : Outport  VectorParamsAs1DForOutWhenUnconnected=off
  Alarm : Outport  Port=2  VectorParamsAs1DForOutWhenUnconnected=off
  wires:
  Compare To Constant/1 -> Alarm/1
  Add3/1 -> Saturation/1
  Constant1/1 -> Add3/1
  Delay/1 -> Add3/3
  Residue/1 -> Add3/2
  Saturation/1 -> CUSUM/1, Delay/1, Compare To Constant/1

== system B20_ATMD_Earthquake/CUSUM/CUSUM_Y6 ==
  Residue : Inport
  Add3 : Sum  Inputs=-++
  Compare To Constant : simulink/Logic and Bit Operations/Compare To Constant  relop=>  const=threshold(i)  OutDataTypeStr=boolean
  Constant1 : Constant  Value=discount(i)
  Delay : Delay  DelayLength=1  SampleTime=Ts
  Saturation : Saturate  UpperLimit=10000  LowerLimit=0
  CUSUM : Outport  VectorParamsAs1DForOutWhenUnconnected=off
  Alarm : Outport  Port=2  VectorParamsAs1DForOutWhenUnconnected=off
  wires:
  Compare To Constant/1 -> Alarm/1
  Add3/1 -> Saturation/1
  Constant1/1 -> Add3/1
  Delay/1 -> Add3/3
  Residue/1 -> Add3/2
  Saturation/1 -> CUSUM/1, Delay/1, Compare To Constant/1

== system B20_ATMD_Earthquake/CUSUM/CUSUM_Y7 ==
  Residue : Inport
  Add3 : Sum  Inputs=-++
  Compare To Constant : simulink/Logic and Bit Operations/Compare To Constant  relop=>  const=threshold(i)  OutDataTypeStr=boolean
  Constant1 : Constant  Value=discount(i)
  Delay : Delay  DelayLength=1  SampleTime=Ts
  Saturation : Saturate  UpperLimit=10000  LowerLimit=0
  CUSUM : Outport  VectorParamsAs1DForOutWhenUnconnected=off
  Alarm : Outport  Port=2  VectorParamsAs1DForOutWhenUnconnected=off
  wires:
  Saturation/1 -> Compare To Constant/1, Delay/1, CUSUM/1
  Residue/1 -> Add3/2
  Delay/1 -> Add3/3
  Constant1/1 -> Add3/1
  Add3/1 -> Saturation/1
  Compare To Constant/1 -> Alarm/1

== system B20_ATMD_Earthquake/CUSUM/CUSUM_Y8 ==
  Residue : Inport
  Add3 : Sum  Inputs=-++
  Compare To Constant : simulink/Logic and Bit Operations/Compare To Constant  relop=>  const=threshold(i)  OutDataTypeStr=boolean
  Constant1 : Constant  Value=discount(i)
  Delay : Delay  DelayLength=1  SampleTime=Ts
  Saturation : Saturate  UpperLimit=10000  LowerLimit=0
  CUSUM : Outport  VectorParamsAs1DForOutWhenUnconnected=off
  Alarm : Outport  Port=2  VectorParamsAs1DForOutWhenUnconnected=off
  wires:
  Saturation/1 -> Compare To Constant/1, Delay/1, CUSUM/1
  Residue/1 -> Add3/2
  Delay/1 -> Add3/3
  Constant1/1 -> Add3/1
  Add3/1 -> Saturation/1
  Compare To Constant/1 -> Alarm/1

== system B20_ATMD_Earthquake/CUSUM/CUSUM_Y9 ==
  Residue : Inport
  Add3 : Sum  Inputs=-++
  Compare To Constant : simulink/Logic and Bit Operations/Compare To Constant  relop=>  const=threshold(i)  OutDataTypeStr=boolean
  Constant1 : Constant  Value=discount(i)
  Delay : Delay  DelayLength=1  SampleTime=Ts
  Saturation : Saturate  UpperLimit=10000  LowerLimit=0
  CUSUM : Outport  VectorParamsAs1DForOutWhenUnconnected=off
  Alarm : Outport  Port=2  VectorParamsAs1DForOutWhenUnconnected=off
  wires:
  Compare To Constant/1 -> Alarm/1
  Add3/1 -> Saturation/1
  Constant1/1 -> Add3/1
  Delay/1 -> Add3/3
  Residue/1 -> Add3/2
  Saturation/1 -> CUSUM/1, Delay/1, Compare To Constant/1

== matlab function B20_ATMD_Earthquake/Subsystem2/Envelope Function ==
  data: u input; y output; t input
function y = fcn(u,t)
%#codegen
t1=6; % 3seconds
t2 =15;
gam=0.26;
if t <= t1
    a = (t/t1)^2; 
    y=a*u;
elseif t >= t1 && t <= t2
    a = 1 ;
    y=a*u;
elseif t > t2
    a = exp(-gam.*(t-t2));
    y= a*u;
else
    y=0*u;
end
end
